simulink model "LFC_two_area_PI_controller"  (R2014a)
settings: Solver=ode45  StartTime=0.0  StopTime=50  RelTol=1e-3
libraries: cstblocks x6
settings Model: Creator=Divya M  LastModifiedBy=Divya M

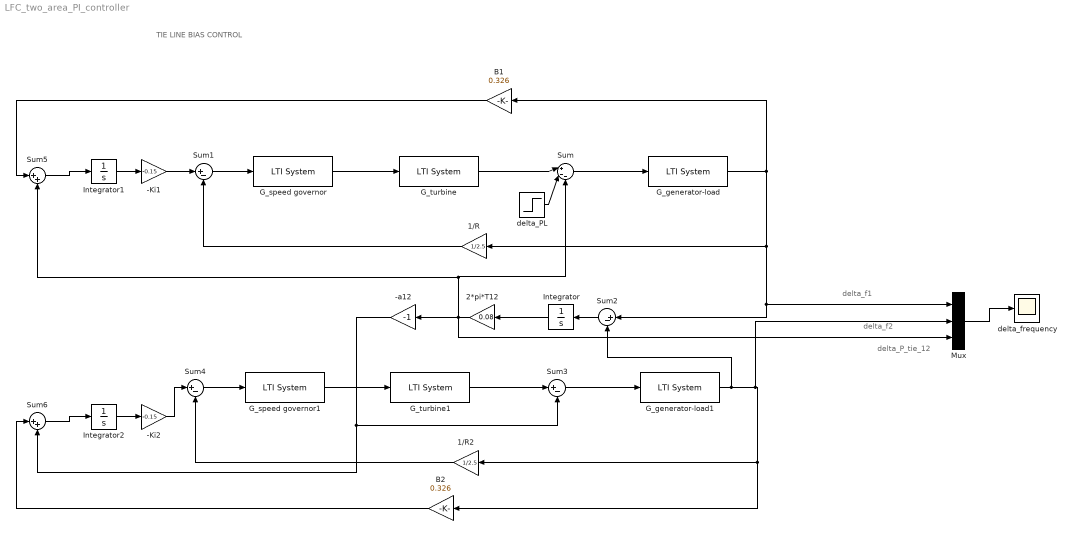
== system LFC_two_area_PI_controller ==
  note: TIE LINE BIAS CONTROL
  note: delta_P_tie_12
  note: delta_f2
  note: delta_f1
  -Ki1 : Gain  Gain=-0.15
  -Ki2 : Gain  Gain=-0.15
  -a12 : Gain  Gain=-1
  1/R : Gain  Gain=1/2.5
  1/R2 : Gain  Gain=1/2.5
  2*pi*T12 : Gain  Gain=0.08
  B1 : Gain  Gain=0.326
  B2 : Gain  Gain=0.326
  G_generator-load : cstblocks/LTI System  sys=tf(105,[22 1])  IC=[]
  G_generator-load1 : cstblocks/LTI System  sys=tf(105,[22 1])  IC=[]
  G_speed governor : cstblocks/LTI System  sys=tf(1,[0.3 1])  IC=[]
  G_speed governor1 : cstblocks/LTI System  sys=tf(1,[0.3 1])  IC=[]
  G_turbine : cstblocks/LTI System  sys=tf(1,[0.5 1])  IC=[]
  G_turbine1 : cstblocks/LTI System  sys=tf(1,[0.5 1])  IC=[]
  Integrator : Integrator
  Integrator1 : Integrator
  Integrator2 : Integrator
  Mux : Mux  Inputs=3
  Sum : Sum  Inputs=|+--
  Sum{1..4} (4 alike) : Sum  Inputs=|+-
  Sum5 : Sum  Inputs=|++
  Sum6 : Sum  Inputs=|++
  delta_PL : Step  After=0.02  SampleTime=0
  delta_frequency : Scope
      settings: YMin=-0.07000000000000001  YMax=0.005
  wires:
  Sum1/1 -> G_speed governor/1
  G_speed governor/1 -> G_turbine/1
  G_turbine/1 -> Sum/1
  Sum/1 -> G_generator-load/1
  G_generator-load/1 -> Sum2/1, Mux/1, 1/R/1, B1/1
  delta_PL/1 -> Sum/2
  1/R/1 -> Sum1/2
  Mux/1 -> delta_frequency/1
  Sum2/1 -> Integrator/1
  Integrator/1 -> 2*pi*T12/1
  2*pi*T12/1 -> Mux/3, -a12/1, Sum5/2, Sum/3
  Sum4/1 -> G_speed governor1/1
  G_speed governor1/1 -> G_turbine1/1
  G_turbine1/1 -> Sum3/1
  Sum3/1 -> G_generator-load1/1
  G_generator-load1/1 -> Mux/2, B2/1, 1/R2/1, Sum2/2
  1/R2/1 -> Sum4/2
  -a12/1 -> Sum6/2, Sum3/2
  Sum5/1 -> Integrator1/1
  -Ki1/1 -> Sum1/1
  Integrator1/1 -> -Ki1/1
  B1/1 -> Sum5/1
  Sum6/1 -> Integrator2/1
  Integrator2/1 -> -Ki2/1
  -Ki2/1 -> Sum4/1
  B2/1 -> Sum6/1
